simulink model "antiresetwindup_control101"  (R2024a)
settings: Solver=VariableStepAuto  StartTime=0.0  StopTime=endtime  RelTol=1e-3
undefined symbols (not defined in the file or in its folder): gamma, umax, umin
libraries: cstblocks x2
settings Model: Creator=barsr  LastModifiedBy=Anthony Rossiter
settings RTWCC: GPUComputeCapability=3.5

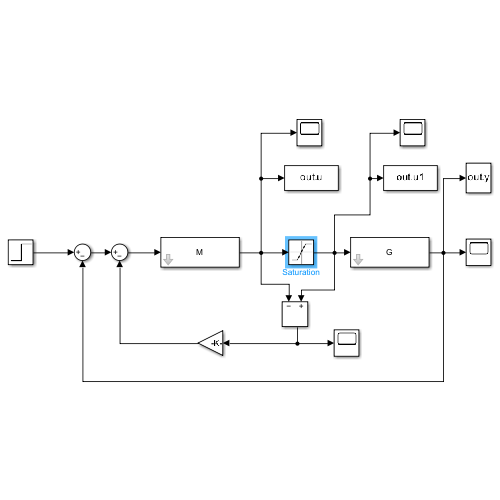
[thumbnail: Simulink's stored preview of the top-level diagram]
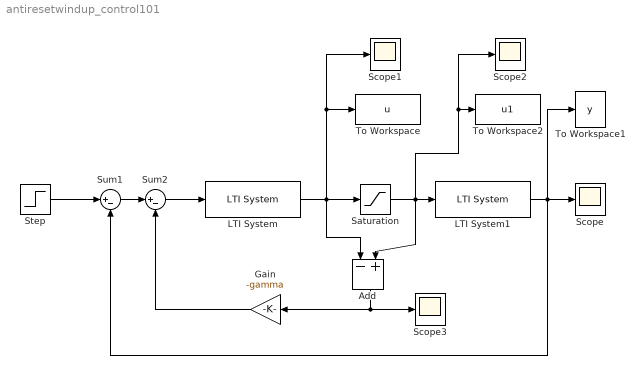
== system antiresetwindup_control101 ==
  Add : Sum  Inputs=-+
  Gain : Gain  Gain=-gamma
  LTI System : cstblocks/LTI System  sys=M  IC=[]  PadeOrder=0
  LTI System1 : cstblocks/LTI System  sys=G  IC=[]  PadeOrder=0
  Saturation : Saturate  UpperLimit=umax  LowerLimit=umin
  Scope{,1..3} (4 alike) : Scope
  Step : Step  Time=0  SampleTime=0
  Sum1 : Sum  Inputs=|+-
  Sum2 : Sum  Inputs=|+-
  To Workspace : ToWorkspace  VariableName=u  SaveFormat=Structure With Time  SampleTime=-1
  To Workspace1 : ToWorkspace  VariableName=y  SaveFormat=Structure With Time  SampleTime=-1
  To Workspace2 : ToWorkspace  VariableName=u1  SaveFormat=Structure With Time  SampleTime=-1
  wires:
  LTI System1/1 -> To Workspace1/1, Sum1/2, Scope/1
  Step/1 -> Sum1/1
  LTI System/1 -> Scope1/1, To Workspace/1, Add/1, Saturation/1
  Saturation/1 -> Add/2, To Workspace2/1, Scope2/1, LTI System1/1
  Add/1 -> Scope3/1, Gain/1
  Gain/1 -> Sum2/2
  Sum1/1 -> Sum2/1
  Sum2/1 -> LTI System/1
